simulink model "double_dm"  (R2023a)
settings: Solver=VariableStepAuto  StartTime=0.0  StopTime=10.0  RelTol=1e-3
settings Model: Creator=isaac  LastModifiedBy=isaac
settings OptimizationCC: ReuseModelBlockBuffer=off

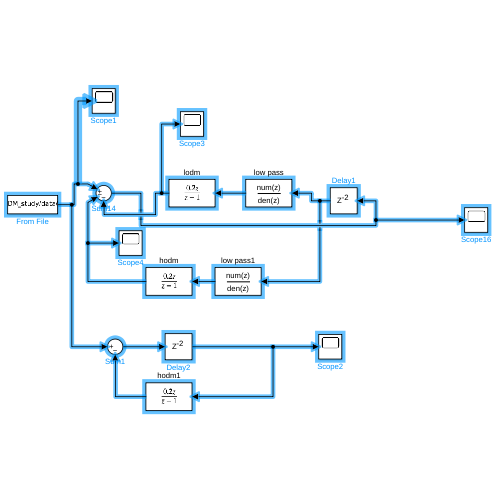
[thumbnail: Simulink's stored preview of the top-level diagram]
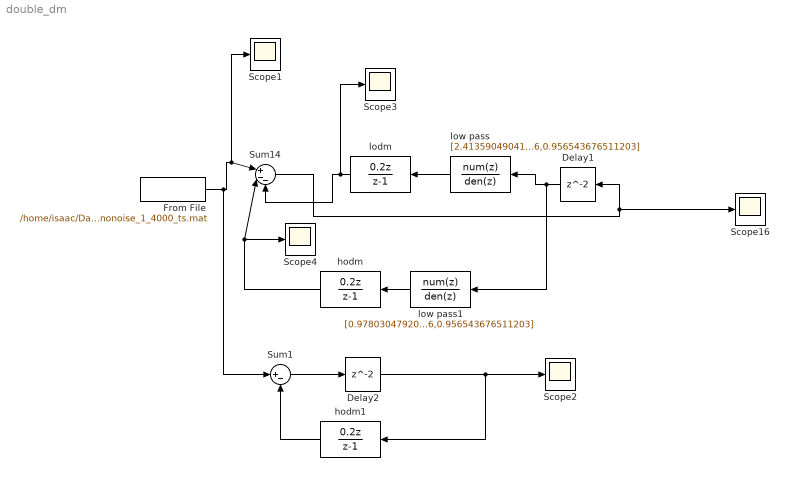
== system double_dm ==
  Delay1 : Delay  SampleTime=0.001
  Delay2 : Delay  SampleTime=0.001
  From File : FromFile  FileName=/home/isaac/Data-Driven-Control-for-AO/2DM_study/data/single_mode_dist_nonoise_1_4000_ts.mat  SampleTime=1/4000
  Scope{1..4,16} (5 alike) : Scope
  Sum1 : Sum  Inputs=|+-
  Sum14 : Sum  Inputs=|+--
  hodm : DiscreteTransferFcn  Numerator=[0.2 0]  Denominator=[1 -1]  SampleTime=0.001
  hodm1 : DiscreteTransferFcn  Numerator=[0.2 0]  Denominator=[1 -1]  SampleTime=0.001
  lodm : DiscreteTransferFcn  Numerator=[0.2 0]  Denominator=[1 -1]  SampleTime=0.001
  low pass : DiscreteFilter  Numerator=[2.413590490419827e-04,4.827180980839655e-04,2.413590490419827e-04]  Denominator=[1,-1.955578240315036,0.956543676511203]  SampleTime=1/2000
  low pass1 : DiscreteFilter  Numerator=[0.978030479206560,-1.956060958413119,0.978030479206560]  Denominator=[1,-1.955578240315036,0.956543676511203]  SampleTime=1/2000
  wires:
  From File/1 -> Sum1/1, Scope1/1, Sum14/1
  low pass1/1 -> hodm/1
  Sum14/1 -> Delay1/1, Scope16/1
  Delay1/1 -> low pass1/1, low pass/1
  low pass/1 -> lodm/1
  lodm/1 -> Scope3/1, Sum14/3
  Delay2/1 -> hodm1/1, Scope2/1
  hodm1/1 -> Sum1/2
  Sum1/1 -> Delay2/1
  hodm/1 -> Sum14/2, Scope4/1
